simulink model "BLAC1_Gradino"  (R2018b)
settings: Solver=ode4  StartTime=0.0  StopTime=0.5  FixedStep=fixed_step_size  MaxStep=.1*Tc  RelTol=1e-4  AbsTol=1e-4
values from neighbouring files (symbols this model uses):
  A1 = -krs*Rs/Lsd    (= -200)    [BLAC1_v1.m]    (also in BLAC1_v2.m; CAE_14_v1.M; CAE_14d.m)
  A10 = -B/(kj*J)    (= 0)    [BLAC1_v1.m]    (also in BLAC1_v2.m; CAE_14_v1.M; CAE_14d.m)
  A11 = -np/(kj*J)    (= -4000)    [BLAC1_v1.m]    (also in BLAC1_v2.m; CAE_14_v1.M; CAE_14d.m)
  A2 = Lsq/Lsd    (= 1)    [BLAC1_v1.m]    (also in BLAC1_v2.m; CAE_14_v1.M; CAE_14d.m)
  A3 = 1/Lsd    (= 200)    [BLAC1_v1.m]    (also in BLAC1_v2.m; CAE_14_v1.M; CAE_14d.m)
  A4 = -Lsd/Lsq    (= -1)    [BLAC1_v1.m]    (also in BLAC1_v2.m; CAE_14_v1.M; CAE_14d.m)
  A5 = -krs*Rs/Lsq    (= -200)    [BLAC1_v1.m]    (also in BLAC1_v2.m; CAE_14_v1.M; CAE_14d.m)
  A6 = -2*Kc*klambda/ms/np/Lsq    (= -20)    [BLAC1_v1.m]    (also in BLAC1_v2.m; CAE_14_v1.M; CAE_14d.m)
  A7 = 1/Lsq    (= 200)    [BLAC1_v1.m]    (also in BLAC1_v2.m; CAE_14_v1.M; CAE_14d.m)
  A8 = Kc*klambda*np/(kj*J)    (= 2400)    [BLAC1_v1.m]    (also in BLAC1_v2.m; CAE_14_v1.M; CAE_14d.m)
  A9 = ms*np^2*(Lsd-Lsq)/2/(kj*J)    (= 0)    [BLAC1_v1.m]    (also in BLAC1_v2.m; CAE_14_v1.M; CAE_14d.m)
  Cr0 = 0    [BLAC0_v1.m]    (also in BLAC1_v1.m; BLAC1_v2.m; CAE_11_v_1.m; CAE_14_v1.M)
  Crn = 0.6    [BLAC0_v1.m]    (also in BLAC1_v1.m; BLAC1_v2.m; CAE_11_v_1.m; CAE_14_v1.M)
  isd0 = 0    [BLAC1_v1.m]    (also in BLAC1_v2.m; CAE_14_v1.M; CAE_14d.m)
  isq0 = (-A10*wdq0-A11*Cr0)/(A8+A9*isd0)    (= 0)    [BLAC1_v1.m]    (also in BLAC1_v2.m; CAE_14_v1.M; CAE_14d.m)
  Kc = ms*np*lambdaf/2    (= 0.27)    [BLAC0_v1.m]    (also in BLAC1_v1.m = 0.6; BLAC1_v2.m = 0.6; CAE_11_v_1.m = 0.6; CAE_14_v1.M = 0.6)
  kf = .1    (= 0.1)    [BLAC1_v1.m]    (also in BLAC1_v2.m; CAE_14_v1.M; CAE_14d.m)
  kiisd = kpisd/tiisd    (= 5000)    [BLAC1_v1.m]    (also in BLAC1_v2.m = kpisd/tiisd; CAE_14_v1.M = kpisd/tiisd; CAE_14d.m = kpisd/tiisd)
  kiisq = kpisq/tiisq    (= 5000)    [BLAC1_v1.m]    (also in BLAC1_v2.m = kpisq/tiisq; CAE_14_v1.M = kpisq/tiisq; CAE_14d.m = kpisq/tiisq)
  kiwr = kpwr/tiw    (= 1.53837822936)    [BLAC1_v1.m]    (also in BLAC1_v2.m; CAE_14_v1.M; CAE_14d.m)
  kpisd = tiisd*Rs/(kf*Tx)    (= 27.8)    [BLAC1_v1.m]    (also in BLAC1_v2.m = tiisd*Rs/(kA*kf*Tx); CAE_14_v1.M = tiisd*Rs/(kA*kf*Tx); CAE_14d.m = tiisd*Rs/(kA*kf*Tx))
  kpisq = tiisq*Rs/(kf*Tx)    (= 27.8)    [BLAC1_v1.m]    (also in BLAC1_v2.m = tiisq*Rs/(kA*kf*Tx); CAE_14_v1.M = tiisq*Rs/(kA*kf*Tx); CAE_14d.m = tiisq*Rs/(kA*kf*Tx))
  kpwr = J*kf/(kT*np*Kc*2*tsigmaw)    (= 0.0113224637681)    [BLAC1_v1.m]    (also in BLAC1_v2.m; CAE_14_v1.M; CAE_14d.m)
  kT = 1    [BLAC1_v1.m]    (also in BLAC1_v2.m; CAE_14_v1.M; CAE_14d.m)
  lambdam = 0.1    [BLAC1_v1.m]    (also in BLAC1_v2.m; CAE_11_v_1.m; CAE_14_v1.M; CAE_14d.m)
  Lsd = 0.005/2    (= 0.0025)    [BLAC0_v1.m]    (also in BLAC1_v1.m = 0.005; BLAC1_v2.m = 0.005; CAE_11_v_1.m = 0.005; CAE_14_v1.M = 0.005)
  Lsq = Lsd    (= 0.0025)    [BLAC0_v1.m]    (also in BLAC1_v1.m = 0.005; BLAC1_v2.m = 0.005; CAE_11_v_1.m = 0.005; CAE_14_v1.M = 0.005)
  ms = 3    [BLAC0_v1.m]    (also in BLAC1_v1.m; BLAC1_v2.m; CAE_11_v_1.m; CAE_14_v1.M)
  np = 2    [BLAC0_v1.m]    (also in BLAC1_v1.m = 4; BLAC1_v2.m = 4; CAE_11_v_1.m = 4; CAE_14_v1.M = 4)
  ppr = 5000    [BLAC1_v1.m]    (also in BLAC1_v2.m; CAE_14_v1.M; CAE_14d.m)
  tA = Tc/2    (= 0.0001)    [BLAC1_v1.m]    (also in BLAC1_v2.m; CAE_14_v1.M; CAE_14d.m)
  tauf = 160e-6    (= 0.00016)    [BLAC1_v1.m]
  taut = 160e-6    (= 0.00016)    [BLAC1_v1.m]
  Tc = 1e-4    (= 0.0001)    [BLAC0_v1.m]    (also in BLAC1_v1.m = 0.0002; BLAC1_v2.m = 0.0002; CAE_14_v1.M = 0.0002; CAE_14d.m = 0.0002)
  tetadq0 = 0    [BLAC1_v1.m]    (also in BLAC1_v2.m; CAE_14_v1.M; CAE_14d.m)
  tsm = tsigmaw*4*1.2    (= 0.008832)    [BLAC1_v2.m]    (also in CAE_14_v1.M; CAE_14d.m)
  wdq0 = 0    [BLAC1_v1.m]    (also in BLAC1_v2.m; CAE_14_v1.M; CAE_14d.m)
  wr0 = 0    [BLAC1_v1.m]    (also in BLAC1_v2.m; CAE_11_v_1.m; CAE_14_v1.M; CAE_14d.m)
  wrr = 1256.6    [BLAC0_v1.m]    (also in BLAC1_v1.m = 300; BLAC1_v2.m = 300)
settings Model: ExtModeTrigMode=oneshot  ExtModeArmWhenConnect=off  Creator=cupertinof  LastModifiedBy=anton
settings SolverCC: AutoScaleAbsTol=off
settings DataIOCC: SaveFormat=Array  SignalLoggingSaveFormat=ModelDataLogs  SaveOutput=off  SaveTime=off  SignalLoggingName=sigsOut
settings OptimizationCC: BooleanDataType=off  ConditionallyExecuteInputs=off  InitFltsAndDblsToZero=on  LifeSpan=inf
settings DebuggingCC: SaveWithParameterizedLinksMsg=none  UnderspecifiedInitializationDetection=Classic  MergeDetectMultiDrivingBlocksExec=none  SignalResolutionControl=TryResolveAllWithWarning  MultiTaskDSMMsg=warning  MultiTaskCondExecSysMsg=none  FcnCallInpInsideContextMsg=warning  StateNameClashWarn=warning  SFUnexpectedBacktrackingDiag=warning  SFNoUnconditionalDefaultTransitionDiag=warning  SFExecutionAtInitializationDiag=none
settings HardwareCC: ProdBitPerPointer=32  ProdBitPerSizeT=32  ProdBitPerPtrDiffT=32  ProdLargestAtomicFloat=None  ProdIntDivRoundTo=Undefined  ProdEndianess=Unspecified  ProdWordSize=32  ProdHWDeviceType=32-bit Generic  TargetUnknown=on
settings ModelReferenceCC: PropagateSignalLabelsOutOfModel=off
settings CodeAppCC: StateflowObjectComments=on
settings GRTTargetCC: TargetFcnLib=ansi_tfl_tmw.mat  TargetLangStandard=C89/C90 (ANSI)  CombineOutputUpdateFcns=off  GRTInterface=on
settings ConfigComp: CovMetricSettings=dw  CovHtmlReporting=on  CovSaveCumulativeToWorkspaceVar=on  CovSaveSingleToWorkspaceVar=on

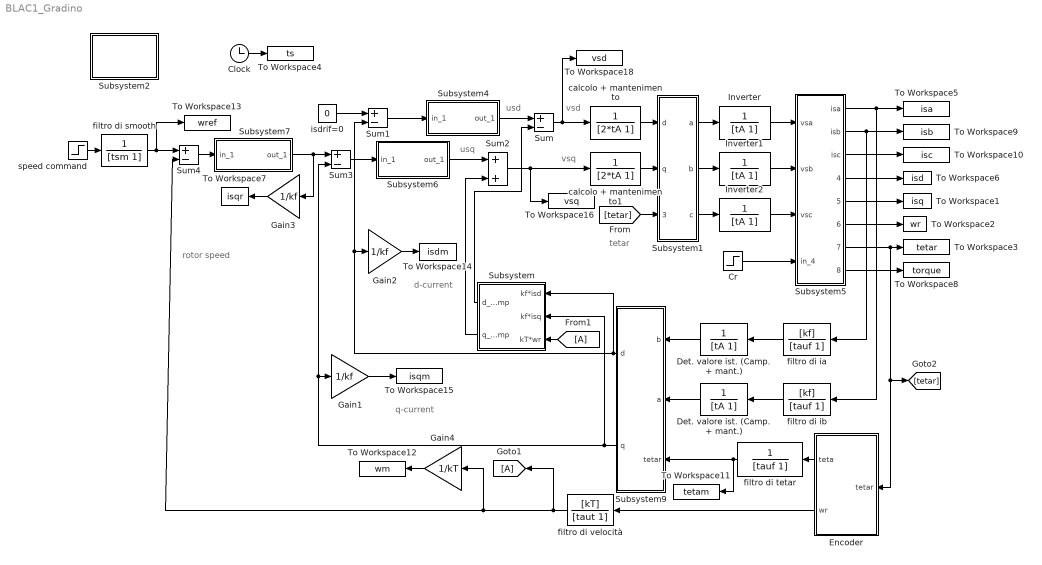
== system BLAC1_Gradino ==
  note: rotor speed
  note: usq
  note: usd
  note: q-current
  note: tetar
  note: vsd
  note: vsq
  note: d-current
  Clock : Clock
  Cr : Step  Time=0.3  Before=Cr0  After=Crn  SampleTime=0
  Det. valore ist. (Camp. + mant.) : TransferFcn  Denominator=[tA 1]
  "Det. valore ist. (Camp. + mant.) " : TransferFcn  Denominator=[tA 1]
  Encoder : Subsystem
  Gain1 : Gain  Gain=1/kf  SaturateOnIntegerOverflow=on  OutDataTypeStr=Inherit: Same as input  ParamDataTypeStr=Inherit: Same as input
  Gain2 : Gain  Gain=1/kf  SaturateOnIntegerOverflow=on  OutDataTypeStr=Inherit: Same as input  ParamDataTypeStr=Inherit: Same as input
  Gain3 : Gain  Gain=1/kf  SaturateOnIntegerOverflow=on  OutDataTypeStr=Inherit: Same as input  ParamDataTypeStr=Inherit: Same as input
  Gain4 : Gain  Gain=1/kT  SaturateOnIntegerOverflow=on  OutDataTypeStr=Inherit: Same as input  ParamDataTypeStr=Inherit: Same as input
  Inverter : TransferFcn  Denominator=[tA 1]
  Inverter1 : TransferFcn  Denominator=[tA 1]
  Inverter2 : TransferFcn  Denominator=[tA 1]
  Subsystem : Subsystem
      mask Display: disp('Decoupling\nNetwork')
  Subsystem1 : Subsystem
      mask Display: disp('d-q\n\na-b-c')
  Subsystem2 : Subsystem
      settings: OpenFcn=BLAC_1d
      mask Display: disp('Load\ndata')
  Subsystem4 : Subsystem
      mask Display: disp('d-current\ncontroller')
  Subsystem5 : Subsystem
      mask Display: disp('BLAC')
  Subsystem6 : Subsystem
      mask Display: disp('q-current\ncontroller')
  Subsystem7 : Subsystem
      mask Display: disp('Speed \ncontroller')
  Subsystem9 : Subsystem
      mask Display: disp('a-b-c\n\nd-q')
  Sum{,1,3..4} (4 alike) : Sum  Inputs=+-  SaturateOnIntegerOverflow=on  InputSameDT=on  OutDataTypeStr=Inherit: Same as first input
  Sum2 : Sum  SaturateOnIntegerOverflow=on  InputSameDT=on  OutDataTypeStr=Inherit: Same as first input
  To Workspace1 : ToWorkspace  VariableName=isq
      settings: MaxDataPoints=1e6
      settings: OpenFcn=|
      | figure(5);
      | plot(ts,isq,'k',ts,isqr,'--k','linewidth',2);
      | xlabel('time [s]');
      | ylabel('isq [A]');title('BLAC motor q-current')
  To Workspace10 : ToWorkspace  VariableName=isc
      settings: OpenFcn=figure(4);plot(ts,isc);xlabel('time [s]');ylabel('isc [A]');title('BLAC motor phase current')  MaxDataPoints=1e6
  To Workspace11 : ToWorkspace  VariableName=tetam
  To Workspace12 : ToWorkspace  VariableName=wm
  To Workspace13 : ToWorkspace  VariableName=wref
  To Workspace14 : ToWorkspace  VariableName=isdm
  To Workspace15 : ToWorkspace  VariableName=isqm
  To Workspace16 : ToWorkspace  VariableName=vsq
  To Workspace18 : ToWorkspace  VariableName=vsd
  To Workspace2 : ToWorkspace  VariableName=wr
      settings: MaxDataPoints=1e6
      settings: OpenFcn=|
      | figure(1);
      | plot(ts,wref,'--k',ts,wr,'k','linewidth',2);
      | xlabel('time [s]');
      | ylabel('speed [rad/s]');
      | title('BLAC motor speed response')
  To Workspace3 : ToWorkspace  VariableName=tetar
  To Workspace4 : ToWorkspace  VariableName=ts
  To Workspace5 : ToWorkspace  VariableName=isa
      settings: OpenFcn=figure(2);plot(ts,isa);xlabel('time [s]');ylabel('isa [A]');title('BLAC motor phase current')  MaxDataPoints=1e6
  To Workspace6 : ToWorkspace  VariableName=isd
      settings: MaxDataPoints=1e6
      settings: OpenFcn=|
      | figure(5);plot(ts,isd,'linewidth',2);xlabel('time [s]');ylabel('isd [A]');title('BLAC motor d-current')
      | axis([0 0.5 -5 20])
  To Workspace7 : ToWorkspace  VariableName=isqr
      settings: OpenFcn=figure(5);plot(ts,isq);xlabel('time [s]');ylabel('isq [A]');title('BLAC motor q-current')  MaxDataPoints=1e6
  To Workspace8 : ToWorkspace  VariableName=torque
      settings: MaxDataPoints=1e6
      settings: OpenFcn=|
      | figure(7);plot(ts,torque,'k','linewidth',2);
      | xlabel('time [s]');
      | ylabel('Electromagnetic torque [Nm]');
      | title('BLAC motor electromagnetic torque')
  To Workspace9 : ToWorkspace  VariableName=isb
      settings: OpenFcn=figure(3);plot(ts,isb);xlabel('time [s]');ylabel('isb [A]');title('BLAC motor phase current')  MaxDataPoints=1e6
  calcolo + mantenimento : TransferFcn  Denominator=[2*tA 1]
  calcolo + mantenimento1 : TransferFcn  Denominator=[2*tA 1]
  filtro di tetar : TransferFcn  Denominator=[tauf 1]
  filtro di smooth : TransferFcn  Denominator=[tsm 1]
  filtro di ia : TransferFcn  Numerator=[kf]  Denominator=[tauf 1]
  filtro di ib : TransferFcn  Numerator=[kf]  Denominator=[tauf 1]
  filtro di velocità : TransferFcn  Numerator=[kT]  Denominator=[taut 1]
  isdrif=0 : Constant  Value=0
  speed command : Step  Time=0.02  Before=wr0*kT  After=wrr*kT  SampleTime=0
  wires:
  Sum3/1 -> Subsystem6/1(in_1)
  Sum4/1 -> Subsystem7/1(in_1)
  Sum/1 -> calcolo + mantenimento/1, To Workspace18/1
  isdrif=0/1 -> Sum1/1
  Sum2/1 -> calcolo + mantenimento1/1, To Workspace16/1
  speed command/1 -> filtro di smooth/1
  Subsystem1/1(a) -> Inverter/1
  Subsystem1/2(b) -> Inverter1/1
  Subsystem1/3(c) -> Inverter2/1
  Subsystem5/8(out_7 1) -> To Workspace8/1
  Subsystem5/6(out_6) -> To Workspace2/1
  Subsystem5/7("out_7 ") -> To Workspace3/1, [tetar], Encoder/1(tetar)
  Subsystem5/4(out_4) -> To Workspace6/1
  Subsystem9/1(d) -> Subsystem/1(kf*isd), Sum1/2, Gain2/1
  Subsystem5/5(out_5) -> To Workspace1/1
  Subsystem9/2(q) -> Subsystem/2(kf*isq), Sum3/2, Gain1/1
  Subsystem4/1(out_1) -> Sum/1
  Subsystem6/1(out_1) -> Sum2/1
  Clock/1 -> To Workspace4/1
  Subsystem5/3(isc) -> To Workspace10/1
  Subsystem5/2(isb) -> To Workspace9/1, filtro di ia/1
  Subsystem5/1(isa) -> To Workspace5/1, filtro di ib/1
  "Det. valore ist. (Camp. + mant.) "/1 -> Subsystem9/1(b)
  Det. valore ist. (Camp. + mant.)/1 -> Subsystem9/2(a)
  calcolo + mantenimento/1 -> Subsystem1/1(d)
  calcolo + mantenimento1/1 -> Subsystem1/2(q)
  Sum1/1 -> Subsystem4/1(in_1)
  Inverter1/1 -> Subsystem5/2(vsb)
  Inverter2/1 -> Subsystem5/3(vsc)
  [tetar] -> Subsystem1/3(tetar)
  Subsystem/1(d_comp) -> Sum/2
  Encoder/1(teta) -> filtro di tetar/1
  Encoder/2(wr) -> filtro di velocità/1
  [A] -> Subsystem/3(kT*wr)
  filtro di ia/1 -> "Det. valore ist. (Camp. + mant.) "/1
  filtro di ib/1 -> Det. valore ist. (Camp. + mant.)/1
  filtro di tetar/1 -> Subsystem9/3(tetar), To Workspace11/1
  Subsystem7/1(out_1) -> Sum3/1, Gain3/1
  filtro di smooth/1 -> Sum4/1, To Workspace13/1
  Cr/1 -> Subsystem5/4(in_4)
  Inverter/1 -> Subsystem5/1(vsa)
  Gain1/1 -> To Workspace15/1
  Gain2/1 -> To Workspace14/1
  Gain3/1 -> To Workspace7/1
  Subsystem/2(q_comp) -> Sum2/2
  filtro di velocità/1 -> [A], Gain4/1, Sum4/2
  Gain4/1 -> To Workspace12/1

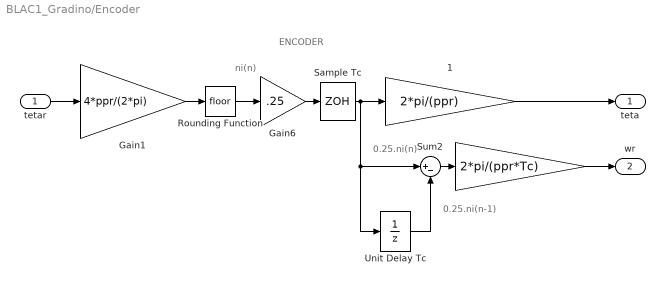
== system BLAC1_Gradino/Encoder ==
  note: ENCODER
  note: 0.25.ni(n-1)
  note: 0.25.ni(n)
  note: ni(n)
  tetar : Inport
  " " : Gain  Gain=2*pi/(ppr*Tc)  SaturateOnIntegerOverflow=on  OutDataTypeStr=Inherit: Same as input  ParamDataTypeStr=Inherit: Same as input
  " 1" : Gain  Gain=2*pi/(ppr)  SaturateOnIntegerOverflow=on  OutDataTypeStr=Inherit: Same as input  ParamDataTypeStr=Inherit: Same as input
  Gain1 : Gain  Gain=4*ppr/(2*pi)  SaturateOnIntegerOverflow=on  OutDataTypeStr=Inherit: Same as input  ParamDataTypeStr=Inherit: Same as input
  Gain6 : Gain  Gain=.25  SaturateOnIntegerOverflow=on  OutDataTypeStr=Inherit: Same as input  ParamDataTypeStr=Inherit: Same as input
  Rounding Function : Rounding
  Sample Tc : ZeroOrderHold  SampleTime=Tc
  Sum2 : Sum  Inputs=|+-  SaturateOnIntegerOverflow=on  InputSameDT=on  OutDataTypeStr=Inherit: Same as first input
  Unit Delay Tc : UnitDelay  SampleTime=Tc
  teta : Outport
  wr : Outport  Port=2
  wires:
  " 1"/1 -> teta/1
  Sum2/1 -> " "/1
  Unit Delay Tc/1 -> Sum2/2
  " "/1 -> wr/1
  Sample Tc/1 -> " 1"/1, Sum2/1, Unit Delay Tc/1
  Rounding Function/1 -> Gain6/1
  tetar/1 -> Gain1/1
  Gain1/1 -> Rounding Function/1
  Gain6/1 -> Sample Tc/1

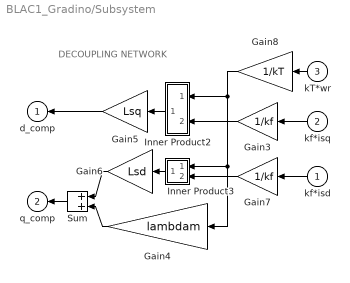
== system BLAC1_Gradino/Subsystem ==
  note: DECOUPLING NETWORK
  kf*isd : Inport
  kf*isq : Inport  Port=2
  kT*wr : Inport  Port=3
  Gain3 : Gain  Gain=1/kf  SaturateOnIntegerOverflow=on  OutDataTypeStr=Inherit: Same as input  ParamDataTypeStr=Inherit: Same as input
  Gain4 : Gain  Gain=lambdam  SaturateOnIntegerOverflow=on  OutDataTypeStr=Inherit: Same as input  ParamDataTypeStr=Inherit: Same as input
  Gain5 : Gain  Gain=Lsq  SaturateOnIntegerOverflow=on  OutDataTypeStr=Inherit: Same as input  ParamDataTypeStr=Inherit: Same as input
  Gain6 : Gain  Gain=Lsd  SaturateOnIntegerOverflow=on  OutDataTypeStr=Inherit: Same as input  ParamDataTypeStr=Inherit: Same as input
  Gain7 : Gain  Gain=1/kf  SaturateOnIntegerOverflow=on  OutDataTypeStr=Inherit: Same as input  ParamDataTypeStr=Inherit: Same as input
  Gain8 : Gain  Gain=1/kT  SaturateOnIntegerOverflow=on  OutDataTypeStr=Inherit: Same as input  ParamDataTypeStr=Inherit: Same as input
  Inner Product2 : Subsystem  mask(Dot Product){}
      mask help:
      | Inner (dot) product.
      | y=sum(u1.*u2)
      mask Help: Computes the inner (dot) product of the inputs: sum(u1.*u2).  The inputs are vectors of the same length. Output is a scalar.
      mask Display: disp('.\n')
  Inner Product3 : Subsystem  mask(Dot Product){}
      mask help:
      | Inner (dot) product.
      | y=sum(u1.*u2)
      mask Help: Computes the inner (dot) product of the inputs: sum(u1.*u2).  The inputs are vectors of the same length. Output is a scalar.
      mask Display: disp('.\n')
  Sum : Sum  SaturateOnIntegerOverflow=on  InputSameDT=on  OutDataTypeStr=Inherit: Same as first input
  d_comp : Outport
  q_comp : Outport  Port=2
  wires:
  Inner Product2/1(out_1) -> Gain5/1
  kf*isq/1 -> Gain3/1
  Inner Product3/1(out_1) -> Gain6/1
  kf*isd/1 -> Gain7/1
  kT*wr/1 -> Gain8/1
  Gain4/1 -> Sum/2
  Gain6/1 -> Sum/1
  Gain5/1 -> d_comp/1
  Sum/1 -> q_comp/1
  Gain3/1 -> Inner Product2/2(in_2)
  Gain7/1 -> Inner Product3/2(in_2)
  Gain8/1 -> Inner Product2/1(in_1), Inner Product3/1(in_1), Gain4/1

== system BLAC1_Gradino/Subsystem1 ==
  d : Inport
  q : Inport  Port=2
  tetar : Inport  Port=3
  Subsystem1 : Subsystem
      mask Display: disp('d,q\n\nalfa,beta')
  Subsystem3 : Subsystem
      mask Display: disp('alfa,beta\na,b,c')
  a : Outport
  b : Outport  Port=2
  c : Outport  Port=3
  wires:
  Subsystem1/2(beta) -> Subsystem3/2(beta)
  Subsystem1/1(alfa) -> Subsystem3/1(alfa)
  d/1 -> Subsystem1/1(d)
  Subsystem3/1(a) -> a/1
  Subsystem3/2(b) -> b/1
  q/1 -> Subsystem1/2(q)
  Subsystem3/3("c ") -> c/1
  tetar/1 -> Subsystem1/3("tetar ")

== system BLAC1_Gradino/Subsystem2 ==

== system BLAC1_Gradino/Subsystem4 ==
  in_1 : Inport
  Gain1 : Gain  Gain=kpisd  SaturateOnIntegerOverflow=on  OutDataTypeStr=Inherit: Same as input  ParamDataTypeStr=Inherit: Same as input
  Gain4 : Gain  Gain=kiisd  SaturateOnIntegerOverflow=on  OutDataTypeStr=Inherit: Same as input  ParamDataTypeStr=Inherit: Same as input
  Integrator1 : Integrator
  Sum2 : Sum  SaturateOnIntegerOverflow=on  InputSameDT=on  OutDataTypeStr=Inherit: Same as first input
  out_1 : Outport
  wires:
  Integrator1/1 -> Sum2/2
  in_1/1 -> Gain1/1, Gain4/1
  Gain1/1 -> Sum2/1
  Sum2/1 -> out_1/1
  Gain4/1 -> Integrator1/1

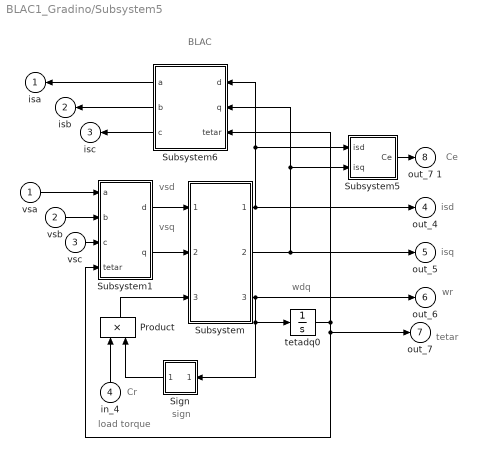
== system BLAC1_Gradino/Subsystem5 ==
  note: wdq
  note: Ce
  note: sign
  note: vsq
  note: vsd
  note: wr
  note: isq
  note: isd
  note: Cr
  note: load torque
  note: BLAC
  note: tetar
  vsa : Inport
  vsb : Inport  Port=2
  vsc : Inport  Port=3
  in_4 : Inport  Port=4
  Product : Product  SaturateOnIntegerOverflow=on  InputSameDT=on  OutDataTypeStr=Inherit: Same as first input
  Sign : Subsystem  mask(Sign){}
      mask help: y = sign(x)
      mask Help: Sign Function:\n\t\t\ty = 1 if x > 0\n\t\t\ty = 0 if x = 0\n\t\t\ty = -1 if x < 0
      mask Display: plot(-50,-50,50,50,[-50,50],[0,0],[0,0],[-50,50],[-40,0],[-30,-30],[0,40],[30,30])
  Subsystem : Subsystem
      mask Display: disp('BLAC\nd-q')
  Subsystem1 : Subsystem
      mask Display: disp('a-b-c\n\nd-q')
  Subsystem5 : Subsystem
      mask Display: disp('Torque')
  Subsystem6 : Subsystem
      mask Display: disp('d-q\n\na-b-c')
  tetadq0 : Integrator  InitialCondition=tetadq0
  isa : Outport
  isb : Outport  Port=2
  isc : Outport  Port=3
  out_4 : Outport  Port=4
  out_5 : Outport  Port=5
  out_6 : Outport  Port=6
  "out_7 " : Outport  Port=7
  out_7 1 : Outport  Port=8
  wires:
  Product/1 -> Subsystem/3(Inport2)
  in_4/1 -> Product/1
  Sign/1(out_1) -> Product/2
  Subsystem/3(Outport2) -> Sign/1(in_1), tetadq0/1, out_6/1
  Subsystem5/1(Ce) -> out_7 1/1
  Subsystem/2(Outport1) -> Subsystem5/2(isq), Subsystem6/2(q), out_5/1
  Subsystem/1(Outport) -> Subsystem5/1(isd), Subsystem6/1(d), out_4/1
  tetadq0/1 -> Subsystem1/4(tetar), "out_7 "/1, Subsystem6/3(tetar)
  Subsystem6/1(a) -> isa/1
  Subsystem6/2(b) -> isb/1
  Subsystem6/3(c) -> isc/1
  Subsystem1/1(d) -> Subsystem/1(Inport)
  Subsystem1/2(q) -> Subsystem/2(Inport1)
  vsa/1 -> Subsystem1/1(a)
  vsb/1 -> Subsystem1/2(b)
  vsc/1 -> Subsystem1/3(c)

== system BLAC1_Gradino/Subsystem6 ==
  in_1 : Inport
  Gain1 : Gain  Gain=kpisq  SaturateOnIntegerOverflow=on  OutDataTypeStr=Inherit: Same as input  ParamDataTypeStr=Inherit: Same as input
  Gain4 : Gain  Gain=kiisq  SaturateOnIntegerOverflow=on  OutDataTypeStr=Inherit: Same as input  ParamDataTypeStr=Inherit: Same as input
  Integrator : Integrator
  Sum2 : Sum  SaturateOnIntegerOverflow=on  InputSameDT=on  OutDataTypeStr=Inherit: Same as first input
  out_1 : Outport
  wires:
  Sum2/1 -> out_1/1
  Gain1/1 -> Sum2/1
  in_1/1 -> Gain1/1, Gain4/1
  Gain4/1 -> Integrator/1
  Integrator/1 -> Sum2/2

== system BLAC1_Gradino/Subsystem7 ==
  note: SPEED CONTROLLER
  in_1 : Inport
  Gain1 : Gain  Gain=kpwr  SaturateOnIntegerOverflow=on  OutDataTypeStr=Inherit: Same as input  ParamDataTypeStr=Inherit: Same as input
  Gain4 : Gain  Gain=kiwr  SaturateOnIntegerOverflow=on  OutDataTypeStr=Inherit: Same as input  ParamDataTypeStr=Inherit: Same as input
  Integrator : Integrator  InitialCondition=isq0
  Sum2 : Sum  SaturateOnIntegerOverflow=on  InputSameDT=on  OutDataTypeStr=Inherit: Same as first input
  out_1 : Outport
  wires:
  Gain4/1 -> Integrator/1
  in_1/1 -> Gain1/1, Gain4/1
  Gain1/1 -> Sum2/1
  Sum2/1 -> out_1/1
  Integrator/1 -> Sum2/2

== system BLAC1_Gradino/Subsystem9 ==
  b : Inport
  a : Inport  Port=2
  tetar : Inport  Port=3
  Subsystem3 : Subsystem
      mask Display: disp('a,b,c\n\nalfa,beta')
  Subsystem4 : Subsystem
      mask Display: disp('alfa,beta\n\nd,q')
  Sum : Sum  Inputs=--  SaturateOnIntegerOverflow=on  InputSameDT=on  OutDataTypeStr=Inherit: Same as first input
  d : Outport
  q : Outport  Port=2
  wires:
  Subsystem3/2(beta) -> Subsystem4/2(beta)
  Subsystem3/1(alfa) -> Subsystem4/1(alfa)
  Subsystem4/1(d) -> d/1
  b/1 -> Subsystem3/2(b), Sum/2
  Subsystem4/2(q) -> q/1
  tetar/1 -> Subsystem4/3("tetar ")
  a/1 -> Subsystem3/1(a), Sum/1
  Sum/1 -> Subsystem3/3(c)

== system BLAC1_Gradino/Subsystem/Inner Product2 ==
  in_1 : Inport
  in_2 : Inport  Port=2
  Product : Product  SaturateOnIntegerOverflow=on  InputSameDT=on  OutDataTypeStr=Inherit: Same as first input
  Sum : Sum  Inputs=+  SaturateOnIntegerOverflow=on  InputSameDT=on  OutDataTypeStr=Inherit: Same as first input
  out_1 : Outport
  wires:
  in_2/1 -> Product/2
  in_1/1 -> Product/1
  Product/1 -> Sum/1
  Sum/1 -> out_1/1

== system BLAC1_Gradino/Subsystem/Inner Product3 ==
  in_1 : Inport
  in_2 : Inport  Port=2
  Product : Product  SaturateOnIntegerOverflow=on  InputSameDT=on  OutDataTypeStr=Inherit: Same as first input
  Sum : Sum  Inputs=+  SaturateOnIntegerOverflow=on  InputSameDT=on  OutDataTypeStr=Inherit: Same as first input
  out_1 : Outport
  wires:
  Sum/1 -> out_1/1
  Product/1 -> Sum/1
  in_1/1 -> Product/1
  in_2/1 -> Product/2

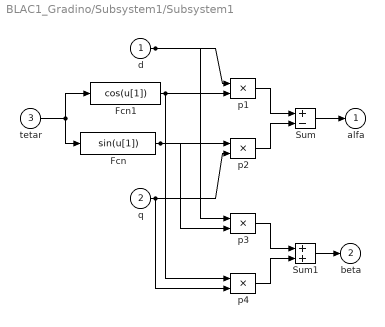
== system BLAC1_Gradino/Subsystem1/Subsystem1 ==
  d : Inport
  q : Inport  Port=2
  "tetar " : Inport  Port=3
  Fcn : Fcn
      mask Display: disp('sin(tetar)')
  Fcn1 : Fcn  Expr=cos(u[1])
      mask Display: disp('cos(tetar)')
  Sum : Sum  Inputs=+-  SaturateOnIntegerOverflow=on  InputSameDT=on  OutDataTypeStr=Inherit: Same as first input
  Sum1 : Sum  SaturateOnIntegerOverflow=on  InputSameDT=on  OutDataTypeStr=Inherit: Same as first input
  p{1..4} (4 alike) : Product  SaturateOnIntegerOverflow=on  InputSameDT=on  OutDataTypeStr=Inherit: Same as first input
  alfa : Outport
  beta : Outport  Port=2
  wires:
  p2/1 -> Sum/2
  p1/1 -> Sum/1
  p3/1 -> Sum1/1
  p4/1 -> Sum1/2
  Sum/1 -> alfa/1
  Sum1/1 -> beta/1
  d/1 -> p1/1, p3/1
  Fcn/1 -> p2/1, p3/2
  q/1 -> p2/2, p4/2
  Fcn1/1 -> p1/2, p4/1
  "tetar "/1 -> Fcn1/1, Fcn/1

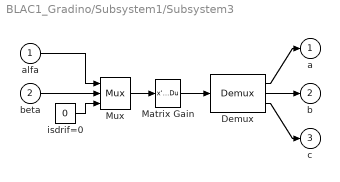
== system BLAC1_Gradino/Subsystem1/Subsystem3 ==
  alfa : Inport
  beta : Inport  Port=2
  Demux : Demux  Outputs=3
  Matrix Gain : StateSpace  A=[]  B=[]  C=[]  D=K  InitialCondition=0  mask(Matrix Gain){K=inv(2/3*[1 -1/2 -1/2;0 sqrt(3)/2 -sqrt(3)/2;1/2 1/2 1/2])}
      mask prompts: K "Gain matrix:"
      mask help: Matrix Gain.
      mask Help: Multiplies input vector by entered matrix to produce output vector (y=Au).
      mask Display: disp('K')
  Mux : Mux  Inputs=3
  isdrif=0 : Constant  Value=0
  a : Outport
  b : Outport  Port=2
  "c " : Outport  Port=3
  wires:
  beta/1 -> Mux/2
  alfa/1 -> Mux/1
  Mux/1 -> Matrix Gain/1
  Matrix Gain/1 -> Demux/1
  Demux/3 -> "c "/1
  Demux/2 -> b/1
  Demux/1 -> a/1
  isdrif=0/1 -> Mux/3

== system BLAC1_Gradino/Subsystem5/Sign ==
  in_1 : Inport
  Constant : Constant  Value=0
  Relational Operator : RelationalOperator  Operator=>  RndMeth=Nearest  InputSameDT=on
  Relational Operator1 : RelationalOperator  Operator=<  RndMeth=Nearest  InputSameDT=on
  Sum : Sum  Inputs=+-  SaturateOnIntegerOverflow=on  InputSameDT=on  OutDataTypeStr=Inherit: Same as first input
  out_1 : Outport
  wires:
  Sum/1 -> out_1/1
  Relational Operator/1 -> Sum/1
  Relational Operator1/1 -> Sum/2
  Constant/1 -> Relational Operator1/2, Relational Operator/2
  in_1/1 -> Relational Operator/1, Relational Operator1/1

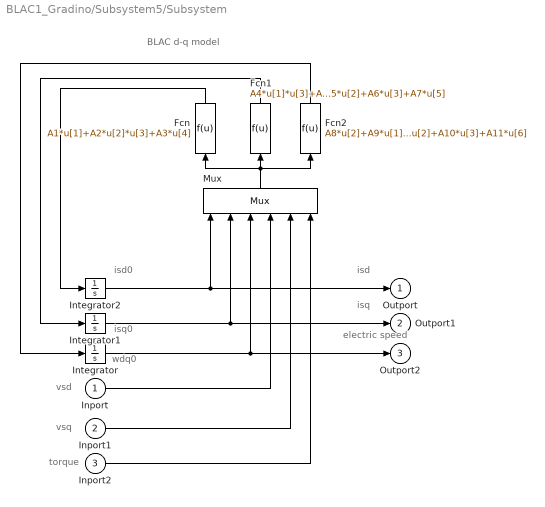
== system BLAC1_Gradino/Subsystem5/Subsystem ==
  note: electric
      | speed
  note: isq
  note: wdq0
  note: isq0
  note: isd0
  note: vsd
  note: isd
  note: torque
  note: vsq
  note: BLAC d-q model
  Inport : Inport
  Inport1 : Inport  Port=2
  Inport2 : Inport  Port=3
  Fcn : Fcn  Expr=A1*u[1]+A2*u[2]*u[3]+A3*u[4]
      mask Display: disp('F1')
  Fcn1 : Fcn  Expr=A4*u[1]*u[3]+A5*u[2]+A6*u[3]+A7*u[5]
      mask Display: disp('F2')
  Fcn2 : Fcn  Expr=A8*u[2]+A9*u[1]*u[2]+A10*u[3]+A11*u[6]
      mask Display: disp('F3')
  Integrator : Integrator  InitialCondition=wdq0
  Integrator1 : Integrator  InitialCondition=isq0
  Integrator2 : Integrator  InitialCondition=isd0
  Mux : Mux  Inputs=6
  Outport : Outport
  Outport1 : Outport  Port=2
  Outport2 : Outport  Port=3
  wires:
  Fcn2/1 -> Integrator/1
  Fcn1/1 -> Integrator1/1
  Fcn/1 -> Integrator2/1
  Mux/1 -> Fcn1/1, Fcn2/1, Fcn/1
  Inport2/1 -> Mux/6
  Inport1/1 -> Mux/5
  Inport/1 -> Mux/4
  Integrator/1 -> Outport2/1, Mux/3
  Integrator1/1 -> Outport1/1, Mux/2
  Integrator2/1 -> Outport/1, Mux/1

== system BLAC1_Gradino/Subsystem5/Subsystem1 ==
  a : Inport
  b : Inport  Port=2
  c : Inport  Port=3
  tetar : Inport  Port=4
  Subsystem3 : Subsystem
      mask Display: disp('a,b,c\n\nalfa,beta')
  Subsystem4 : Subsystem
      mask Display: disp('alfa,beta\n\nd,q')
  d : Outport
  q : Outport  Port=2
  wires:
  Subsystem3/2(beta) -> Subsystem4/2(beta)
  Subsystem3/1(alfa) -> Subsystem4/1(alfa)
  a/1 -> Subsystem3/1(a)
  Subsystem4/1(d) -> d/1
  b/1 -> Subsystem3/2(b)
  c/1 -> Subsystem3/3(c)
  Subsystem4/2(q) -> q/1
  tetar/1 -> Subsystem4/3("tetar ")

== system BLAC1_Gradino/Subsystem5/Subsystem5 ==
  isd : Inport
  isq : Inport  Port=2
  Gain2 : Gain  Gain=ms/2*np*(Lsd-Lsq)  SaturateOnIntegerOverflow=on  OutDataTypeStr=Inherit: Same as input  ParamDataTypeStr=Inherit: Same as input
  Gain3 : Gain  Gain=Kc  SaturateOnIntegerOverflow=on  OutDataTypeStr=Inherit: Same as input  ParamDataTypeStr=Inherit: Same as input
  Product : Product  SaturateOnIntegerOverflow=on  InputSameDT=on  OutDataTypeStr=Inherit: Same as first input
  Sum : Sum  SaturateOnIntegerOverflow=on  InputSameDT=on  OutDataTypeStr=Inherit: Same as first input
  Ce : Outport
  wires:
  isd/1 -> Product/1
  Product/1 -> Gain2/1
  isq/1 -> Product/2, Gain3/1
  Gain3/1 -> Sum/2
  Sum/1 -> Ce/1
  Gain2/1 -> Sum/1

== system BLAC1_Gradino/Subsystem5/Subsystem6 ==
  d : Inport
  q : Inport  Port=2
  tetar : Inport  Port=3
  Subsystem1 : Subsystem
      mask Display: disp('d,q\n\nalfa,beta')
  Subsystem3 : Subsystem
      mask Display: disp('alfa,beta\na,b,c')
  a : Outport
  b : Outport  Port=2
  c : Outport  Port=3
  wires:
  Subsystem1/2(beta) -> Subsystem3/2(beta)
  Subsystem1/1(alfa) -> Subsystem3/1(alfa)
  d/1 -> Subsystem1/1(d)
  Subsystem3/1(a) -> a/1
  Subsystem3/2(b) -> b/1
  q/1 -> Subsystem1/2(q)
  Subsystem3/3("c ") -> c/1
  tetar/1 -> Subsystem1/3("tetar ")

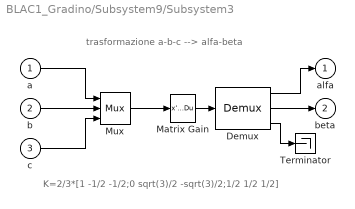
== system BLAC1_Gradino/Subsystem9/Subsystem3 ==
  note: trasformazione a-b-c --> alfa-beta
  note: K=2/3*[1 -1/2 -1/2;0 sqrt(3)/2 -sqrt(3)/2;1/2 1/2 1/2]
  a : Inport
  b : Inport  Port=2
  c : Inport  Port=3
  Demux : Demux  Outputs=3
  Matrix Gain : StateSpace  A=[]  B=[]  C=[]  D=K  InitialCondition=0  mask(Matrix Gain){K=2/3*[1 -1/2 -1/2;0 sqrt(3)/2 -sqrt(3)/2;1/2 1/2 1/2]}
      mask prompts: K "Gain matrix:"
      mask help: Matrix Gain.
      mask Help: Multiplies input vector by entered matrix to produce output vector (y=Au).
      mask Display: disp('K')
  Mux : Mux  Inputs=3
  Terminator : Terminator
  alfa : Outport
  beta : Outport  Port=2
  wires:
  Demux/1 -> alfa/1
  c/1 -> Mux/3
  b/1 -> Mux/2
  a/1 -> Mux/1
  Mux/1 -> Matrix Gain/1
  Matrix Gain/1 -> Demux/1
  Demux/2 -> beta/1
  Demux/3 -> Terminator/1

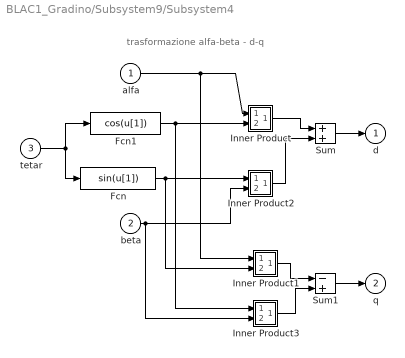
== system BLAC1_Gradino/Subsystem9/Subsystem4 ==
  note: trasformazione alfa-beta - d-q
  alfa : Inport
  beta : Inport  Port=2
  "tetar " : Inport  Port=3
  Fcn : Fcn
      mask Display: disp('sin(tetar)')
  Fcn1 : Fcn  Expr=cos(u[1])
      mask Display: disp('cos(tetar)')
  Inner Product : Subsystem  mask(Dot Product){}
      mask help:
      | Inner (dot) product.
      | y=sum(u1.*u2)
      mask Help: Computes the inner (dot) product of the inputs: sum(u1.*u2).  The inputs are vectors of the same length. Output is a scalar.
      mask Display: disp('.\n')
  Inner Product1 : Subsystem  mask(Dot Product){}
      mask help:
      | Inner (dot) product.
      | y=sum(u1.*u2)
      mask Help: Computes the inner (dot) product of the inputs: sum(u1.*u2).  The inputs are vectors of the same length. Output is a scalar.
      mask Display: disp('.\n')
  Inner Product2 : Subsystem  mask(Dot Product){}
      mask help:
      | Inner (dot) product.
      | y=sum(u1.*u2)
      mask Help: Computes the inner (dot) product of the inputs: sum(u1.*u2).  The inputs are vectors of the same length. Output is a scalar.
      mask Display: disp('.\n')
  Inner Product3 : Subsystem  mask(Dot Product){}
      mask help:
      | Inner (dot) product.
      | y=sum(u1.*u2)
      mask Help: Computes the inner (dot) product of the inputs: sum(u1.*u2).  The inputs are vectors of the same length. Output is a scalar.
      mask Display: disp('.\n')
  Sum : Sum  SaturateOnIntegerOverflow=on  InputSameDT=on  OutDataTypeStr=Inherit: Same as first input
  Sum1 : Sum  Inputs=-+  SaturateOnIntegerOverflow=on  InputSameDT=on  OutDataTypeStr=Inherit: Same as first input
  d : Outport
  q : Outport  Port=2
  wires:
  Inner Product3/1(out_1) -> Sum1/2
  Inner Product1/1(out_1) -> Sum1/1
  Fcn1/1 -> Inner Product/2(in_2), Inner Product3/1(in_1)
  Inner Product2/1(out_1) -> Sum/2
  Inner Product/1(out_1) -> Sum/1
  Sum/1 -> d/1
  Sum1/1 -> q/1
  Fcn/1 -> Inner Product1/2(in_2), Inner Product2/1(in_1)
  alfa/1 -> Inner Product1/1(in_1), Inner Product/1(in_1)
  beta/1 -> Inner Product2/2(in_2), Inner Product3/2(in_2)
  "tetar "/1 -> Fcn1/1, Fcn/1

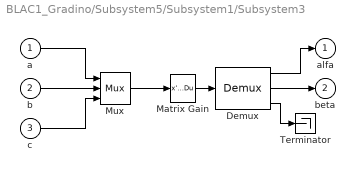
== system BLAC1_Gradino/Subsystem5/Subsystem1/Subsystem3 ==
  a : Inport
  b : Inport  Port=2
  c : Inport  Port=3
  Demux : Demux  Outputs=3
  Matrix Gain : StateSpace  A=[]  B=[]  C=[]  D=K  InitialCondition=0  mask(Matrix Gain){K=2/3*[1 -1/2 -1/2;0 sqrt(3)/2 -sqrt(3)/2;1/2 1/2 1/2]}
      mask prompts: K "Gain matrix:"
      mask help: Matrix Gain.
      mask Help: Multiplies input vector by entered matrix to produce output vector (y=Au).
      mask Display: disp('K')
  Mux : Mux  Inputs=3
  Terminator : Terminator
  alfa : Outport
  beta : Outport  Port=2
  wires:
  Demux/1 -> alfa/1
  c/1 -> Mux/3
  b/1 -> Mux/2
  a/1 -> Mux/1
  Mux/1 -> Matrix Gain/1
  Matrix Gain/1 -> Demux/1
  Demux/2 -> beta/1
  Demux/3 -> Terminator/1

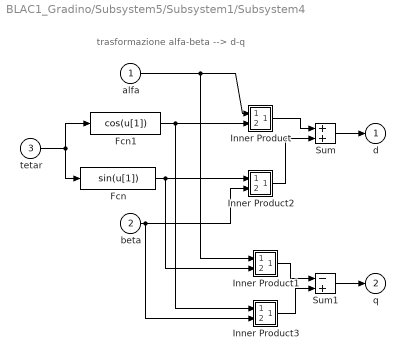
== system BLAC1_Gradino/Subsystem5/Subsystem1/Subsystem4 ==
  note: trasformazione alfa-beta --> d-q
  alfa : Inport
  beta : Inport  Port=2
  "tetar " : Inport  Port=3
  Fcn : Fcn
      mask Display: disp('sin(tetar)')
  Fcn1 : Fcn  Expr=cos(u[1])
      mask Display: disp('cos(tetar)')
  Inner Product : Subsystem  mask(Dot Product){}
      mask help:
      | Inner (dot) product.
      | y=sum(u1.*u2)
      mask Help: Computes the inner (dot) product of the inputs: sum(u1.*u2).  The inputs are vectors of the same length. Output is a scalar.
      mask Display: disp('.\n')
  Inner Product1 : Subsystem  mask(Dot Product){}
      mask help:
      | Inner (dot) product.
      | y=sum(u1.*u2)
      mask Help: Computes the inner (dot) product of the inputs: sum(u1.*u2).  The inputs are vectors of the same length. Output is a scalar.
      mask Display: disp('.\n')
  Inner Product2 : Subsystem  mask(Dot Product){}
      mask help:
      | Inner (dot) product.
      | y=sum(u1.*u2)
      mask Help: Computes the inner (dot) product of the inputs: sum(u1.*u2).  The inputs are vectors of the same length. Output is a scalar.
      mask Display: disp('.\n')
  Inner Product3 : Subsystem  mask(Dot Product){}
      mask help:
      | Inner (dot) product.
      | y=sum(u1.*u2)
      mask Help: Computes the inner (dot) product of the inputs: sum(u1.*u2).  The inputs are vectors of the same length. Output is a scalar.
      mask Display: disp('.\n')
  Sum : Sum  SaturateOnIntegerOverflow=on  InputSameDT=on  OutDataTypeStr=Inherit: Same as first input
  Sum1 : Sum  Inputs=-+  SaturateOnIntegerOverflow=on  InputSameDT=on  OutDataTypeStr=Inherit: Same as first input
  d : Outport
  q : Outport  Port=2
  wires:
  Inner Product3/1(out_1) -> Sum1/2
  Inner Product1/1(out_1) -> Sum1/1
  Fcn1/1 -> Inner Product/2(in_2), Inner Product3/1(in_1)
  Inner Product2/1(out_1) -> Sum/2
  Inner Product/1(out_1) -> Sum/1
  Sum/1 -> d/1
  Sum1/1 -> q/1
  Fcn/1 -> Inner Product1/2(in_2), Inner Product2/1(in_1)
  alfa/1 -> Inner Product1/1(in_1), Inner Product/1(in_1)
  beta/1 -> Inner Product2/2(in_2), Inner Product3/2(in_2)
  "tetar "/1 -> Fcn1/1, Fcn/1

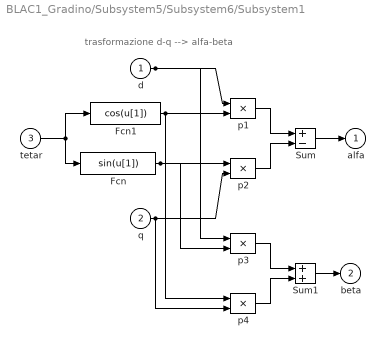
== system BLAC1_Gradino/Subsystem5/Subsystem6/Subsystem1 ==
  note: trasformazione d-q --> alfa-beta
  d : Inport
  q : Inport  Port=2
  "tetar " : Inport  Port=3
  Fcn : Fcn
      mask Display: disp('sin(tetar)')
  Fcn1 : Fcn  Expr=cos(u[1])
      mask Display: disp('cos(tetar)')
  Sum : Sum  Inputs=+-  SaturateOnIntegerOverflow=on  InputSameDT=on  OutDataTypeStr=Inherit: Same as first input
  Sum1 : Sum  SaturateOnIntegerOverflow=on  InputSameDT=on  OutDataTypeStr=Inherit: Same as first input
  p{1..4} (4 alike) : Product  SaturateOnIntegerOverflow=on  InputSameDT=on  OutDataTypeStr=Inherit: Same as first input
  alfa : Outport
  beta : Outport  Port=2
  wires:
  p2/1 -> Sum/2
  p1/1 -> Sum/1
  p3/1 -> Sum1/1
  p4/1 -> Sum1/2
  Sum/1 -> alfa/1
  Sum1/1 -> beta/1
  d/1 -> p1/1, p3/1
  Fcn/1 -> p2/1, p3/2
  q/1 -> p2/2, p4/2
  Fcn1/1 -> p1/2, p4/1
  "tetar "/1 -> Fcn1/1, Fcn/1

== system BLAC1_Gradino/Subsystem5/Subsystem6/Subsystem3 ==
  note: trasformazione alfa-beta --> a-b-c
  note: inv(2/3*[1 -1/2 -1/2;0 sqrt(3)/2 -sqrt(3)/2;1/2 1/2 1/2])
  alfa : Inport
  beta : Inport  Port=2
  Constant : Constant  Value=0
  Demux : Demux  Outputs=3
  Matrix Gain : StateSpace  A=[]  B=[]  C=[]  D=K  InitialCondition=0  mask(Matrix Gain){K=inv(2/3*[1 -1/2 -1/2;0 sqrt(3)/2 -sqrt(3)/2;1/2 1/2 1/2])}
      mask prompts: K "Gain matrix:"
      mask help: Matrix Gain.
      mask Help: Multiplies input vector by entered matrix to produce output vector (y=Au).
      mask Display: disp('K')
  Mux : Mux  Inputs=3
  a : Outport
  b : Outport  Port=2
  "c " : Outport  Port=3
  wires:
  beta/1 -> Mux/2
  alfa/1 -> Mux/1
  Mux/1 -> Matrix Gain/1
  Matrix Gain/1 -> Demux/1
  Demux/3 -> "c "/1
  Demux/2 -> b/1
  Demux/1 -> a/1
  Constant/1 -> Mux/3

== system BLAC1_Gradino/Subsystem9/Subsystem4/Inner Product ==
  in_1 : Inport
  in_2 : Inport  Port=2
  Product : Product  SaturateOnIntegerOverflow=on  InputSameDT=on  OutDataTypeStr=Inherit: Same as first input
  Sum : Sum  Inputs=+  SaturateOnIntegerOverflow=on  InputSameDT=on  OutDataTypeStr=Inherit: Same as first input
  out_1 : Outport
  wires:
  Sum/1 -> out_1/1
  Product/1 -> Sum/1
  in_1/1 -> Product/1
  in_2/1 -> Product/2

== system BLAC1_Gradino/Subsystem9/Subsystem4/Inner Product1 ==
  in_1 : Inport
  in_2 : Inport  Port=2
  Product : Product  SaturateOnIntegerOverflow=on  InputSameDT=on  OutDataTypeStr=Inherit: Same as first input
  Sum : Sum  Inputs=+  SaturateOnIntegerOverflow=on  InputSameDT=on  OutDataTypeStr=Inherit: Same as first input
  out_1 : Outport
  wires:
  in_2/1 -> Product/2
  in_1/1 -> Product/1
  Product/1 -> Sum/1
  Sum/1 -> out_1/1

== system BLAC1_Gradino/Subsystem9/Subsystem4/Inner Product2 ==
  in_1 : Inport
  in_2 : Inport  Port=2
  Product : Product  SaturateOnIntegerOverflow=on  InputSameDT=on  OutDataTypeStr=Inherit: Same as first input
  Sum : Sum  Inputs=+  SaturateOnIntegerOverflow=on  InputSameDT=on  OutDataTypeStr=Inherit: Same as first input
  out_1 : Outport
  wires:
  Sum/1 -> out_1/1
  Product/1 -> Sum/1
  in_1/1 -> Product/1
  in_2/1 -> Product/2

== system BLAC1_Gradino/Subsystem9/Subsystem4/Inner Product3 ==
  in_1 : Inport
  in_2 : Inport  Port=2
  Product : Product  SaturateOnIntegerOverflow=on  InputSameDT=on  OutDataTypeStr=Inherit: Same as first input
  Sum : Sum  Inputs=+  SaturateOnIntegerOverflow=on  InputSameDT=on  OutDataTypeStr=Inherit: Same as first input
  out_1 : Outport
  wires:
  Sum/1 -> out_1/1
  Product/1 -> Sum/1
  in_1/1 -> Product/1
  in_2/1 -> Product/2

== system BLAC1_Gradino/Subsystem5/Subsystem1/Subsystem4/Inner Product ==
  in_1 : Inport
  in_2 : Inport  Port=2
  Product : Product  SaturateOnIntegerOverflow=on  InputSameDT=on  OutDataTypeStr=Inherit: Same as first input
  Sum : Sum  Inputs=+  SaturateOnIntegerOverflow=on  InputSameDT=on  OutDataTypeStr=Inherit: Same as first input
  out_1 : Outport
  wires:
  Sum/1 -> out_1/1
  Product/1 -> Sum/1
  in_1/1 -> Product/1
  in_2/1 -> Product/2

== system BLAC1_Gradino/Subsystem5/Subsystem1/Subsystem4/Inner Product1 ==
  in_1 : Inport
  in_2 : Inport  Port=2
  Product : Product  SaturateOnIntegerOverflow=on  InputSameDT=on  OutDataTypeStr=Inherit: Same as first input
  Sum : Sum  Inputs=+  SaturateOnIntegerOverflow=on  InputSameDT=on  OutDataTypeStr=Inherit: Same as first input
  out_1 : Outport
  wires:
  in_2/1 -> Product/2
  in_1/1 -> Product/1
  Product/1 -> Sum/1
  Sum/1 -> out_1/1

== system BLAC1_Gradino/Subsystem5/Subsystem1/Subsystem4/Inner Product2 ==
  in_1 : Inport
  in_2 : Inport  Port=2
  Product : Product  SaturateOnIntegerOverflow=on  InputSameDT=on  OutDataTypeStr=Inherit: Same as first input
  Sum : Sum  Inputs=+  SaturateOnIntegerOverflow=on  InputSameDT=on  OutDataTypeStr=Inherit: Same as first input
  out_1 : Outport
  wires:
  Sum/1 -> out_1/1
  Product/1 -> Sum/1
  in_1/1 -> Product/1
  in_2/1 -> Product/2

== system BLAC1_Gradino/Subsystem5/Subsystem1/Subsystem4/Inner Product3 ==
  in_1 : Inport
  in_2 : Inport  Port=2
  Product : Product  SaturateOnIntegerOverflow=on  InputSameDT=on  OutDataTypeStr=Inherit: Same as first input
  Sum : Sum  Inputs=+  SaturateOnIntegerOverflow=on  InputSameDT=on  OutDataTypeStr=Inherit: Same as first input
  out_1 : Outport
  wires:
  Sum/1 -> out_1/1
  Product/1 -> Sum/1
  in_1/1 -> Product/1
  in_2/1 -> Product/2
